simulink model "MBD_W3_P2"  (R2020a)
settings: Solver=FixedStepDiscrete  StartTime=0.0  StopTime=150.0  FixedStep=0.1  RelTol=1e-3
undefined symbols (not defined in the file): DiscIntNeverNeededParam
libraries: simulink x1
settings Model: Creator=Atri Mondal  LastModifiedBy=Atri Mondal

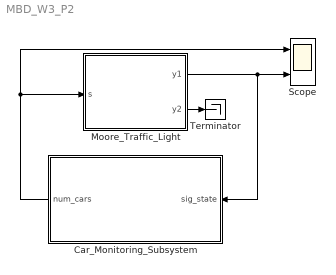
== system MBD_W3_P2 ==
  Car_Monitoring_Subsystem : Subsystem
  Moore_Traffic_Light : Stateflow chart  TreatAsAtomicUnit=on
  Scope : Scope  NumInputPorts=2
  Terminator : Terminator
  wires:
  Moore_Traffic_Light/1(y1) -> Scope/2, Car_Monitoring_Subsystem/1(sig_state)
  Moore_Traffic_Light/2(y2) -> Terminator/1
  Car_Monitoring_Subsystem/1(num_cars) -> Scope/1, Moore_Traffic_Light/1(s)

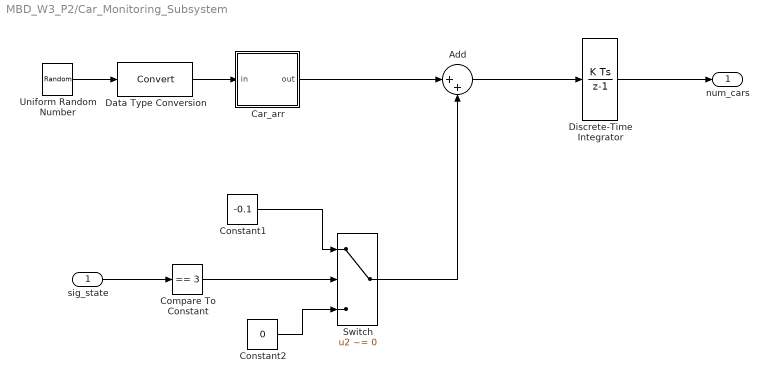
== system MBD_W3_P2/Car_Monitoring_Subsystem ==
  sig_state : Inport
  Add : Sum  Inputs=|++
  Car_arr : Stateflow chart  TreatAsAtomicUnit=on
  Compare To Constant : simulink/Logic and Bit Operations/Compare To Constant  relop===  const=3  OutDataTypeStr=boolean  ZeroCross=off
  Constant1 : Constant  Value=-0.1
  Constant2 : Constant  Value=0
  Data Type Conversion : DataTypeConversion
  Discrete-Time Integrator : DiscreteIntegrator  SampleTime=-1  LimitOutput=on  LowerSaturationLimit=0  ICPrevOutput=DiscIntNeverNeededParam  ICPrevScaledInput=DiscIntNeverNeededParam
  Switch : Switch  Criteria=u2 ~= 0
  Uniform Random Number : UniformRandomNumber  Minimum=0  Maximum=100  Seed=177836  SampleTime=0
  num_cars : Outport  VectorParamsAs1DForOutWhenUnconnected=off
  wires:
  Constant1/1 -> Switch/1
  Constant2/1 -> Switch/3
  Discrete-Time Integrator/1 -> num_cars/1
  sig_state/1 -> Compare To Constant/1
  Compare To Constant/1 -> Switch/2
  Switch/1 -> Add/2
  Add/1 -> Discrete-Time Integrator/1
  Car_arr/1(out) -> Add/1
  Data Type Conversion/1 -> Car_arr/1(in)
  Uniform Random Number/1 -> Data Type Conversion/1

== stateflow chart MBD_W3_P2/Moore_Traffic_Light ==
  settings: stateMachineType=MOORE_MACHINE  executeAtInitialization=1  initializeOutput=1
  state Stop_for_Traffic
    y1 = R;
    y2 = G;
  state Stop
    y1 = R;
    y2 = G;
  state Stop_to_Go
    y1 = R;
    y2 = Y;
  state Go_to_Stop
    y1 = Y;
    y2 = R;
  state Go
    y1 = G;
    y2 = R;
  (default) -> Stop
  Stop_for_Traffic -> Stop_to_Go : [s]
  Stop -> Stop_for_Traffic : after(20,tick)
  Go_to_Stop -> Stop : after (3,tick)
  Stop_to_Go -> Go : after(3,tick)
  Go -> Go_to_Stop : after(10,tick)
  data: s input double; y1 output double; R constant uint8 =1; Y constant double =2; G constant double =3; y2 output double

== stateflow chart MBD_W3_P2/Car_Monitoring_Subsystem/Car_arr ==
  (default) -> (junction 2) : {out = in > 98;}
  data: in input int8; out output double
